simulink model "Stateflow1"  (R2025b)
settings: Solver=FixedStepAuto  StartTime=0.0  StopTime=inf  RelTol=1e-3  EnableMultiTasking=on
libraries: simulink x6, raspberrypiBasiclib x4, raspberrypiNetworklib x1
settings Model: ExtModeTrigDuration=2  Creator=jujma  LastModifiedBy=jujma
settings SolverCC: PositivePriorityOrder=on
settings OptimizationCC: EnhancedBackFolding=on  PassReuseOutputArgsAs=Individual arguments  ZeroExternalMemoryAtStartup=off  ZeroInternalMemoryAtStartup=off  MaxStackSize=200000  OptimizeBlockOrder=speed  DifferentSizesBufferReuse=on  OptimizationCustomize=off  EfficientTunableParamExpr=on
settings DebuggingCC: ParameterTunabilityLossMsg=error
settings HardwareCC: ProdBitPerPointer=32.0  ProdBitPerSizeT=32.0  ProdBitPerPtrDiffT=32.0  ProdLargestAtomicInteger=Long  ProdLargestAtomicFloat=Double  ProdWordSize=32.0  ProdLongLongMode=on  ProdHWDeviceType=ARM Compatible->ARM Cortex-A (32-bit)
settings RTWCC: SystemTargetFile=ert.tlc  HardwareBoard=Raspberry Pi  TLCOptions="-aInlineSetEventsForThisBaseRateFcn=TLC_FALSE -aSuppressMultiTaskScheduler=TLC_FALSE  -aRateBasedStepFcn=0"  TemplateMakefile=ert_default_tmf  Toolchain=GNU GCC Embedded Linux  BuildConfiguration=Faster Runs  Description=Embedded Coder
settings CodeAppCC: ForceParamTrailComments=on  IgnoreCustomStorageClasses=off  OperatorAnnotations=on  SimulinkDataObjDesc=on  SFDataObjDesc=on  InsertBlockDesc=on
settings ERTTargetCC: ExtModeTransport=2.0  ExtModeStaticAlloc=on  ExtModeMexFile=ext_xcp  ExtModeIntrfLevel=Level2 - Open  InlinedParameterPlacement=Hierarchical  CodeReplacementLibrary=ARM Cortex-A CMSIS  SupportVariableSizeSignals=on

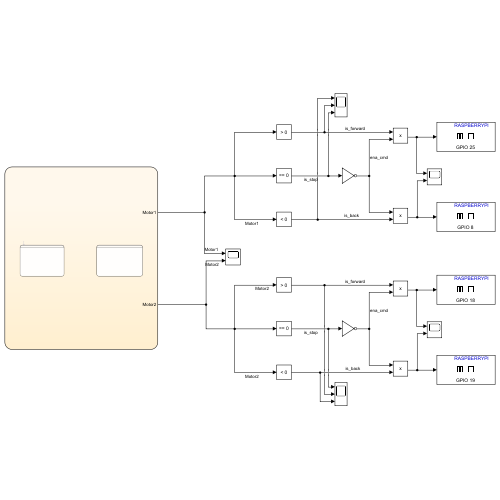
[thumbnail: Simulink's stored preview of the top-level diagram]
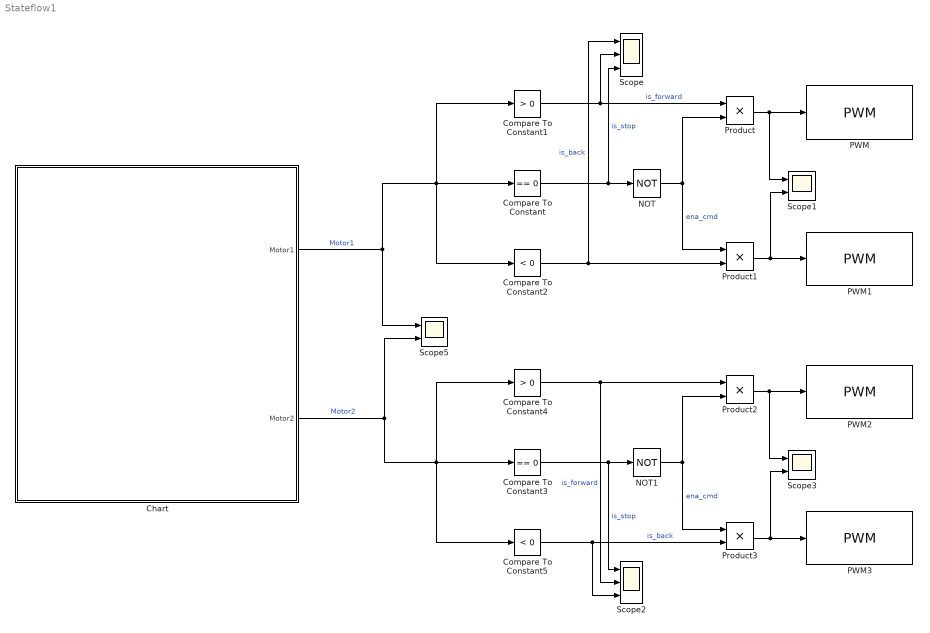
== system Stateflow1 ==
  Chart : Stateflow chart  TreatAsAtomicUnit=on
  Compare To Constant : simulink/Logic and Bit Operations/Compare To Constant  relop===  const=0  OutDataTypeStr=boolean
  Compare To Constant1 : simulink/Logic and Bit Operations/Compare To Constant  relop=>  const=0  OutDataTypeStr=boolean
  Compare To Constant2 : simulink/Logic and Bit Operations/Compare To Constant  relop=<  const=0  OutDataTypeStr=boolean
  Compare To Constant3 : simulink/Logic and Bit Operations/Compare To Constant  relop===  const=0  OutDataTypeStr=boolean
  Compare To Constant4 : simulink/Logic and Bit Operations/Compare To Constant  relop=>  const=0  OutDataTypeStr=boolean
  Compare To Constant5 : simulink/Logic and Bit Operations/Compare To Constant  relop=<  const=0  OutDataTypeStr=boolean
  NOT : Logic  Operator=NOT  IconShape=distinctive  AllPortsSameDT=off  OutDataTypeStr=boolean
  NOT1 : Logic  Operator=NOT  IconShape=distinctive  AllPortsSameDT=off  OutDataTypeStr=boolean
  PWM : raspberrypiBasiclib/PWM  board=Pi Zero W  Pin_=25  Frequency=500  blockPlatform=Raspberry Pi
  PWM1 : raspberrypiBasiclib/PWM  board=Pi Zero W  Pin_=8  Frequency=500  blockPlatform=Raspberry Pi
  PWM2 : raspberrypiBasiclib/PWM  board=Pi Zero W  Pin_=18  Frequency=500  blockPlatform=Raspberry Pi
  PWM3 : raspberrypiBasiclib/PWM  board=Pi Zero W  Pin_=19  Frequency=500  blockPlatform=Raspberry Pi
  Product{,1..3} (4 alike) : Product
  Scope : Scope  NumInputPorts=3
      settings: ActiveDisplayYMinimum=-0.12499999999999997  ActiveDisplayYMaximum=1.125
  Scope1 : Scope  NumInputPorts=2
      settings: ActiveDisplayYMinimum=-16.578406132891736  ActiveDisplayYMaximum=15.421593867108266
  Scope2 : Scope  NumInputPorts=3
      settings: ActiveDisplayYMinimum=-0.12499999999999997  ActiveDisplayYMaximum=1.125  DataLoggingVariableName=ScopeData2
  Scope3 : Scope  NumInputPorts=2
      settings: ActiveDisplayYMinimum=-16.578406132891736  ActiveDisplayYMaximum=15.421593867108266  DataLoggingVariableName=ScopeData3
  Scope5 : Scope  NumInputPorts=2
      settings: ActiveDisplayYMinimum=-1.25  ActiveDisplayYMaximum=1.25  DataLoggingVariableName=ScopeData5
  wires:
  Compare To Constant5/1 -> Scope2/3, Product3/2  "is_back"
  Compare To Constant4/1 -> Scope2/2, Product2/1  "is_forward"
  NOT1/1 -> Product2/2, Product3/1  "ena_cmd"
  Compare To Constant3/1 -> Scope2/1, NOT1/1  "is_stop"
  Product1/1 -> Scope1/2, PWM1/1
  NOT/1 -> Product/2, Product1/1  "ena_cmd"
  Chart/2(Motor2) -> Scope5/2, Compare To Constant4/1, Compare To Constant5/1, Compare To Constant3/1  "Motor2"
  Compare To Constant/1 -> Scope/3, NOT/1  "is_stop"
  Chart/1(Motor1) -> Scope5/1, Compare To Constant1/1, Compare To Constant2/1, Compare To Constant/1  "Motor1"
  Product2/1 -> Scope3/1, PWM2/1
  Product3/1 -> Scope3/2, PWM3/1
  Product/1 -> Scope1/1, PWM/1
  Compare To Constant2/1 -> Scope/1, Product1/2  "is_back"
  Compare To Constant1/1 -> Scope/2, Product/1  "is_forward"

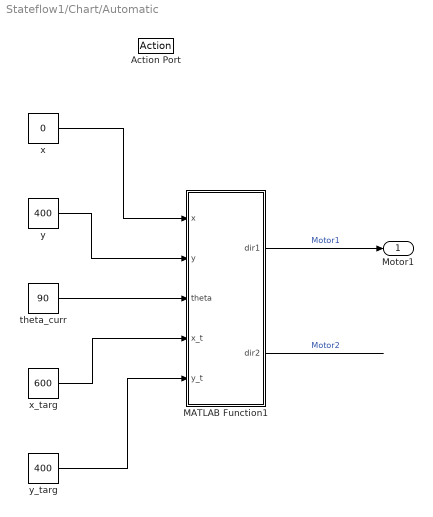
== system Stateflow1/Chart/Automatic ==
  Action Port : ActionPort
      settings: CopyFcn=Stateflow.SLINSF.SimulinkMan.removeBlockPreDeleteFcn  PreDeleteFcn=Stateflow.SLINSF.SimulinkMan.unsafePredeleteFcn
  MATLAB Function1 : MATLAB Function  TreatAsAtomicUnit=on
  theta_curr : Constant  Value=90
  x : Constant  Value=0
  x_targ : Constant  Value=600
  y : Constant  Value=400
  y_targ : Constant  Value=400
  Motor1 : Outport
  wires:
  theta_curr/1 -> MATLAB Function1/3(theta)
  y_targ/1 -> MATLAB Function1/5(y_t)
  y/1 -> MATLAB Function1/2(y)
  x/1 -> MATLAB Function1/1(x)
  x_targ/1 -> MATLAB Function1/4(x_t)
  MATLAB Function1/1(dir1) -> Motor1/1  "Motor1"
  MATLAB Function1/2(dir2) -> ?  "Motor2"

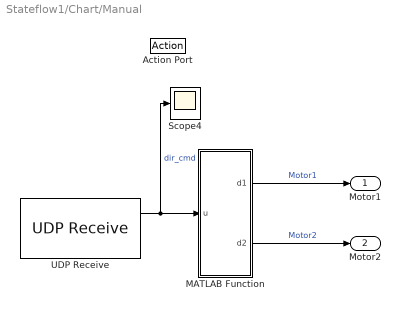
== system Stateflow1/Chart/Manual ==
  Action Port : ActionPort
      settings: CopyFcn=Stateflow.SLINSF.SimulinkMan.removeBlockPreDeleteFcn  PreDeleteFcn=Stateflow.SLINSF.SimulinkMan.unsafePredeleteFcn
  MATLAB Function : MATLAB Function  TreatAsAtomicUnit=on
  Scope4 : Scope
      settings: ActiveDisplayYMinimum=-1.25  ActiveDisplayYMaximum=1.25  DataLoggingVariableName=ScopeData4
  UDP Receive : raspberrypiNetworklib/UDP Receive  localURL='0.0.0.0'  localPort=55001  remoteURL='0.0.0.0'  remotePort=-1  recvBufferSize=8192  signalDatatype=double  dims=2  isVarSize=off  showBlockingTime=off  blockingTime=0  sampletime=0.0001  blockPlatform=Raspberry Pi
  Motor1 : Outport  OutDataTypeStr=double
  Motor2 : Outport  Port=2
  wires:
  UDP Receive/1 -> MATLAB Function/1(u), Scope4/1  "dir_cmd"
  MATLAB Function/2(d2) -> Motor2/1  "Motor2"
  MATLAB Function/1(d1) -> Motor1/1  "Motor1"

== matlab function Stateflow1/Chart/Automatic/MATLAB Function1 ==
  data: x input; dir1 output; y input; theta input; x_t input; y_t input; dir2 output
function [dir1, dir2] = GoToGoal(x, y, theta, x_t, y_t)
% x, y, theta: current pose
% x_t, y_t: target position
% vL, vR: desired left/right wheel linear velocities (0-1)

    % Distance and angle to target
    ex = x_t - x;
    ey = y_t - y;
    d  = sqrt(ex^2 + ey^2);

    % Persistent mode:
    % 1 = rotate to face target
    % 2 = drive straight to target
    persistent mode
    if isempty(mode)
        mode = 1;
    end

    % Tolerances
    d_tol     = 0.02;          % distance tolerance (m)
    angle_tol = 5 * pi / 180;  % angle tolerance (rad), ~5 degrees

    % If already close enough: stop, reset mode, and return
    if d < d_tol
        dir1 = 0;
        dir2 = 0;
        mode = 1;   % next target will start in rotate mode
        return;
    end

    % Desired heading and heading error
    psi     = atan2(ey, ex);          % desired heading
    e_theta = wrapToPi(psi - theta);  % heading error in [-pi, pi]

    switch mode
        case 1  % rotate in place until facing the target
            if abs(e_theta) > angle_tol
                % If error > 0, target is to the "left" → rotate CCW
                if e_theta > 0
                    dir1 = -1;  % left wheel backward
                    dir2 =  1;  % right wheel forward
                else
                    dir1 =  1;  % left wheel forward
                    dir2 = -1;  % right wheel backward
                end
            else
                % Heading good enough: switch to driving straight
                mode = 2;
                dir1 = 1;
                dir2 = 1;
            end

        case 2  % drive straight towards the target
            if d > d_tol
                % Just go straight forward
                dir1 = 1;
                dir2 = 1;
            else
                % Close enough: stop and reset
                dir1 = 0;
                dir2 = 0;
                mode = 1;
            end

        otherwise
            % Safety fallback
            dir1 = 0;
            dir2 = 0;
            mode = 1;
    end
end

function a = wrapToPi(a)
% Wrap angle a to the range (-pi, pi]
    a = mod(a + pi, 2*pi) - pi;
end

== matlab function Stateflow1/Chart/Manual/MATLAB Function ==
  data: u input; d1 output; d2 output
function [d1, d2] = split_cmd(u)
%#codegen
% u is a 1x2 vector: [dir1 dir2]
d1 = u(1);
d2 = u(2);
end

== stateflow chart Stateflow1/Chart ==
  state Manual
  state Automatic
  (default) -> Manual
  data: sf_internal_action_state_placeholder_data local double size=1 =0; sf_internal_action_state_placeholder_data local double size=1 =0; Motor1 output; Motor2 output
